simulink model "svpwm_2level_using_function"  (R2023a)
settings: Solver=VariableStepAuto  StartTime=0.0  StopTime=0.5  RelTol=1e-3
libraries: spsIGBTDiodeLib x6, spsVoltageMeasurementLib x5, spsSeriesRLCBranchLib x3, simulink x1, spsabctoAlphaBetaZeroLib x1, spsDCVoltageSourceLib x1, spsGroundLib x1, sps_lib x1
settings Model: Creator=yadur  LastModifiedBy=yadur

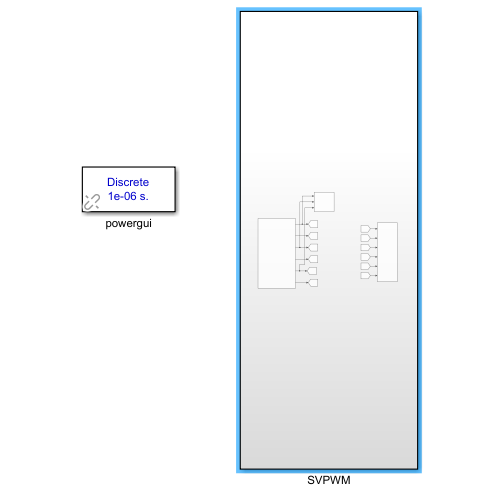
[thumbnail: Simulink's stored preview of the top-level diagram]
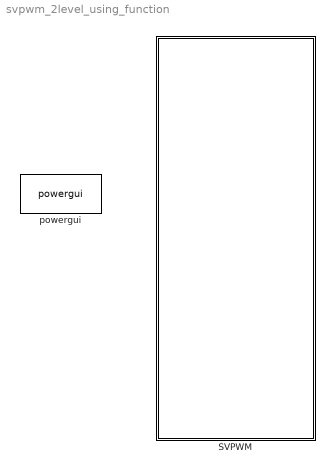
== system svpwm_2level_using_function ==
  SVPWM : Subsystem
  powergui : sps_lib/powergui  Priority=1  SimulationMode=Discrete  SampleTime=1e-6  frequency=60  Iterations=50  frequencyindice=0  Pbase=100e6  ErrMax=1e-4  UnitsV=kV  UnitsW=MW  buscounter=0  FunctionMessages=off  echomessages=off  EnableUseOfTLC=off  CurrentSourceSwitches=off  DisableSnubberDevices=off  DisableRonSwitches=off  DisableVfSwitches=off  DisplayEquations=off  AutomaticDiscreteSolvers=off  SolverType=Tustin/Backward Euler (TBE)  Interpol=off  ExternalGateDelay=off  methode=off  Ts=100  x0status=blocks  SPID=on  SwTol=0  HookPort=off  NonlinearTolerance=1e-4  nMaxIteration=100  ContinueOnMaxIteration=off  RestoreLinks=warning  ResistiveCurrentMeasurement=off  Frange=[0:2:500]  Ylog=off  Xlog=on  ShowGrid=off  save=off  variable=ZData  structure=0  ZoomFFT=off  StartTime=0.0  cycles=1  DisplayStyle=1  fundamental=60  FreqAxis=off  MaxFrequency=1000  frequencyindicesteady=1  RmsSteady=1  display=off

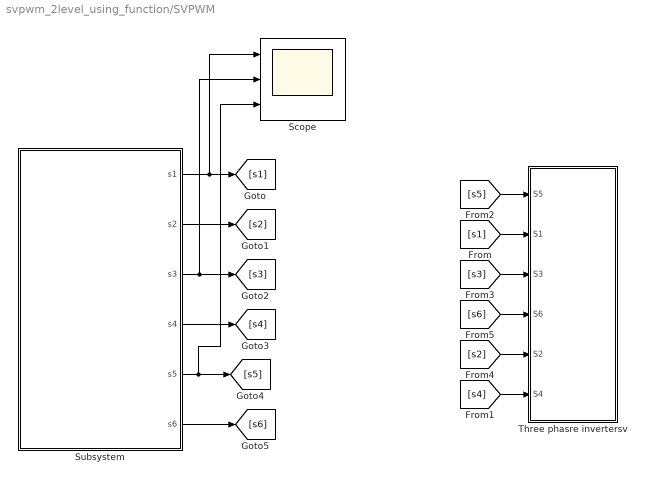
== system svpwm_2level_using_function/SVPWM ==
  Scope : Scope  NumInputPorts=3
  Subsystem : Subsystem
  Three phasre invertersv : Subsystem
  wires:
  [s1] -> Three phasre invertersv/2(S1)
  [s5] -> Three phasre invertersv/1(S5)
  [s3] -> Three phasre invertersv/3(S3)
  [s2] -> Three phasre invertersv/5(S2)
  Subsystem/6(s6) -> [s6]
  [s4] -> Three phasre invertersv/6(S4)
  Subsystem/5(s5) -> Scope/3, [s5]
  [s6] -> Three phasre invertersv/4(S6)
  Subsystem/1(s1) -> Scope/1, [s1]
  Subsystem/2(s2) -> [s2]
  Subsystem/4(s4) -> [s4]
  Subsystem/3(s3) -> Scope/2, [s3]

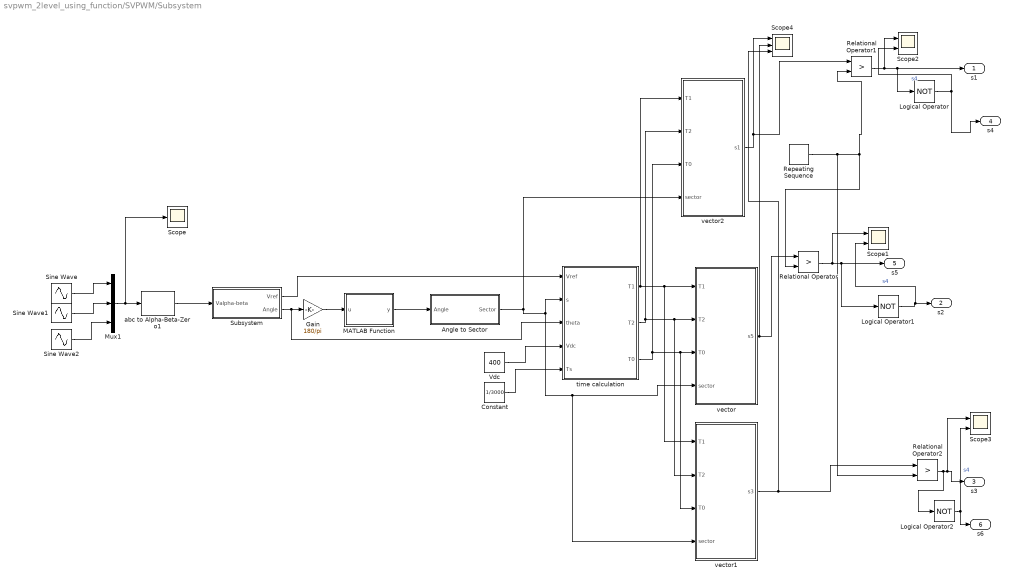
== system svpwm_2level_using_function/SVPWM/Subsystem ==
  Angle to Sector : Subsystem
  Constant : Constant  Value=1/3000
  Gain : Gain  Gain=180/pi
  Logical Operator : Logic  Operator=NOT  AllPortsSameDT=off  OutDataTypeStr=boolean
  Logical Operator1 : Logic  Operator=NOT  AllPortsSameDT=off  OutDataTypeStr=boolean
  Logical Operator2 : Logic  Operator=NOT  AllPortsSameDT=off  OutDataTypeStr=boolean
  MATLAB Function : MATLAB Function  TreatAsAtomicUnit=on
  Mux1 : Mux  Inputs=3
  Relational Operator : RelationalOperator  Operator=>  OutDataTypeStr=boolean  RndMeth=Simplest  InputSameDT=off
  Relational Operator1 : RelationalOperator  Operator=>  OutDataTypeStr=boolean  RndMeth=Simplest  InputSameDT=off
  Relational Operator2 : RelationalOperator  Operator=>  OutDataTypeStr=boolean  RndMeth=Simplest  InputSameDT=off
  Repeating Sequence : simulink/Sources/Repeating Sequence  rep_seq_t="[0  1]*[1/3000]"  rep_seq_y=[0 0.0025]
  Scope : Scope
  Scope1 : Scope  NumInputPorts=2
  Scope2 : Scope  NumInputPorts=2
  Scope3 : Scope  NumInputPorts=2
  Scope4 : Scope  NumInputPorts=3
  Sine Wave : Sin  Amplitude=230  Frequency=2*pi*50  SampleTime=0
  Sine Wave1 : Sin  Amplitude=230  Frequency=2*pi*50  Phase=2*pi/3  SampleTime=0
  Sine Wave2 : Sin  Amplitude=230  Frequency=2*pi*50  Phase=4*pi/3  SampleTime=0
  Subsystem : Subsystem
  Vdc : Constant  Value=400
  abc to Alpha-Beta-Zero1 : spsabctoAlphaBetaZeroLib/abc to Alpha-Beta-Zero
  time calculation : MATLAB Function  TreatAsAtomicUnit=on
  vector : MATLAB Function  TreatAsAtomicUnit=on
  vector1 : MATLAB Function  TreatAsAtomicUnit=on
  vector2 : MATLAB Function  TreatAsAtomicUnit=on
  s1 : Outport
  s2 : Outport  Port=2
  s3 : Outport  Port=3
  s4 : Outport  Port=4
  s5 : Outport  Port=5
  s6 : Outport  Port=6
  wires:
  Angle to Sector/1(Sector) -> vector1/4(sector), vector/4(sector), time calculation/2(s), vector2/4(sector)
  Sine Wave1/1 -> Mux1/2
  abc to Alpha-Beta-Zero1/1 -> Subsystem/1(Valpha-beta)
  Mux1/1 -> Scope/1, abc to Alpha-Beta-Zero1/1
  Vdc/1 -> time calculation/4(Vdc)
  Sine Wave/1 -> Mux1/1
  time calculation/3(T0) -> vector2/3(T0), vector1/3(T0), vector/3(T0)
  time calculation/1(T1) -> vector2/1(T1), vector1/1(T1), vector/1(T1)
  time calculation/2(T2) -> vector1/2(T2), vector/2(T2), vector2/2(T2)
  Logical Operator/1 -> s4/1, Scope2/2  "s4"
  Sine Wave2/1 -> Mux1/3
  vector/1(s5) -> Scope4/2, Relational Operator/1
  Relational Operator/1 -> Scope1/1, Logical Operator1/1, s5/1
  Relational Operator1/1 -> Scope2/1, Logical Operator/1, s1/1
  vector2/1(s1) -> Scope4/1, Relational Operator1/1
  Repeating Sequence/1 -> Relational Operator2/2, Relational Operator1/2, Relational Operator/2
  Relational Operator2/1 -> Logical Operator2/1, Scope3/1, s3/1
  vector1/1(s3) -> Scope4/3, Relational Operator2/1
  Logical Operator1/1 -> Scope1/2, s2/1  "s4"
  Logical Operator2/1 -> s6/1, Scope3/2  "s4"
  Constant/1 -> time calculation/5(Ts)
  Subsystem/1(Vref) -> time calculation/1(Vref)
  Subsystem/2(Angle) -> time calculation/3(theta), Gain/1
  Gain/1 -> MATLAB Function/1(u)
  MATLAB Function/1(y) -> Angle to Sector/1(Angle)

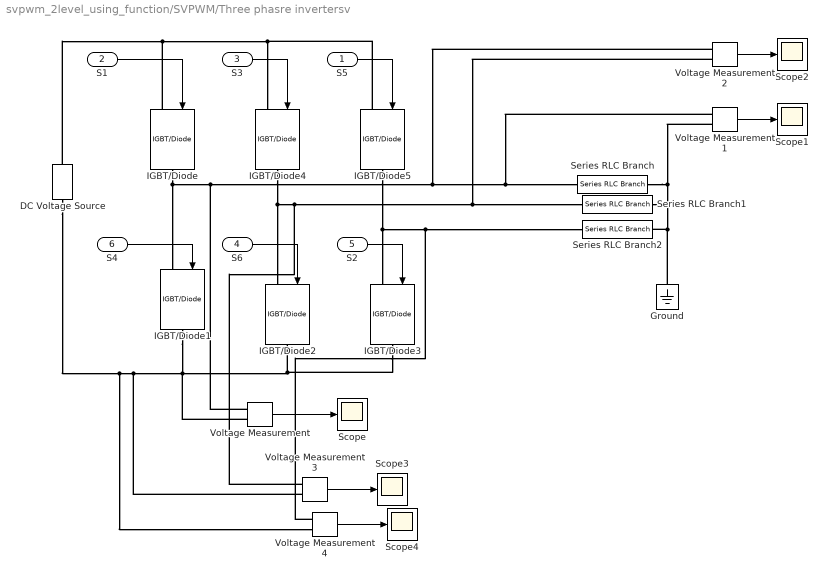
== system svpwm_2level_using_function/SVPWM/Three phasre invertersv ==
  S5 : Inport
  S1 : Inport  Port=2
  S3 : Inport  Port=3
  S6 : Inport  Port=4
  S2 : Inport  Port=5
  S4 : Inport  Port=6
  DC Voltage Source : spsDCVoltageSourceLib/DC Voltage Source  Amplitude=400  Measurements=None
  Ground : spsGroundLib/Ground  LConnTagsString=a
  IGBT/Diode{,1..5} (6 alike) : spsIGBTDiodeLib/IGBT//Diode  Ron=1e-3  Rs=1e5  Cs=inf  Measurements=off
  Scope{,1..4} (5 alike) : Scope
  Series RLC Branch : spsSeriesRLCBranchLib/Series RLC Branch  LConnTagsString=__new0  RConnTagsString=__new0  BranchType=R  Resistance=1  Inductance=1e-3  SetiL0=off  InitialCurrent=0  Capacitance=1e-6  Setx0=off  InitialVoltage=0  Measurements=None
  Series RLC Branch1 : spsSeriesRLCBranchLib/Series RLC Branch  LConnTagsString=__new0  RConnTagsString=__new0  BranchType=R  Resistance=1  Inductance=1e-3  SetiL0=off  InitialCurrent=0  Capacitance=1e-6  Setx0=off  InitialVoltage=0  Measurements=None
  Series RLC Branch2 : spsSeriesRLCBranchLib/Series RLC Branch  LConnTagsString=__new0  RConnTagsString=__new0  BranchType=R  Resistance=1  Inductance=1e-3  SetiL0=off  InitialCurrent=0  Capacitance=1e-6  Setx0=off  InitialVoltage=0  Measurements=None
  Voltage Measurement{,1..4} (5 alike) : spsVoltageMeasurementLib/Voltage Measurement  PhasorSimulation=off  OutputType=Complex  PSBequivalent=0
  wires:
  Voltage Measurement1/1 -> Scope1/1
  Voltage Measurement/1 -> Scope/1
  Voltage Measurement2/1 -> Scope2/1
  S3/1 -> IGBT/Diode4/1
  S5/1 -> IGBT/Diode5/1
  S2/1 -> IGBT/Diode3/1
  S4/1 -> IGBT/Diode1/1
  S6/1 -> IGBT/Diode2/1
  S1/1 -> IGBT/Diode/1
  Voltage Measurement3/1 -> Scope3/1
  Voltage Measurement4/1 -> Scope4/1
  connections:
  IGBT/Diode3/RConn1 -- IGBT/Diode2/RConn1 -- Voltage Measurement3/LConn2 -- Voltage Measurement4/LConn2 -- DC Voltage Source/LConn1 -- Voltage Measurement/LConn2 -- IGBT/Diode1/RConn1
  IGBT/Diode5/RConn1 -- IGBT/Diode3/LConn1 -- Voltage Measurement4/LConn1 -- Series RLC Branch2/LConn1
  IGBT/Diode5/LConn1 -- DC Voltage Source/RConn1 -- IGBT/Diode/LConn1 -- IGBT/Diode4/LConn1
  IGBT/Diode4/RConn1 -- IGBT/Diode2/LConn1 -- Voltage Measurement3/LConn1 -- Voltage Measurement2/LConn2 -- Series RLC Branch1/LConn1
  IGBT/Diode/RConn1 -- Voltage Measurement/LConn1 -- Voltage Measurement2/LConn1 -- Voltage Measurement1/LConn1 -- Series RLC Branch/LConn1 -- IGBT/Diode1/LConn1
  Series RLC Branch/RConn1 -- Ground/LConn1 -- Series RLC Branch2/RConn1 -- Series RLC Branch1/RConn1 -- Voltage Measurement1/LConn2

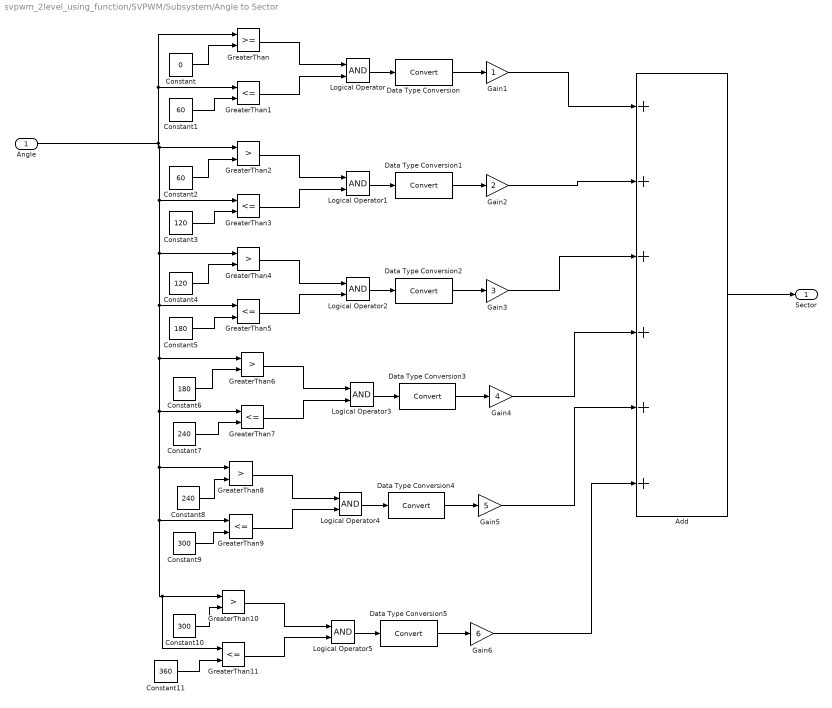
== system svpwm_2level_using_function/SVPWM/Subsystem/Angle to Sector ==
  Angle : Inport
  Add : Sum  Inputs=++++++
  Constant : Constant  Value=0
  Constant1 : Constant  Value=60
  Constant10 : Constant  Value=300
  Constant11 : Constant  Value=360
  Constant2 : Constant  Value=60
  Constant3 : Constant  Value=120
  Constant4 : Constant  Value=120
  Constant5 : Constant  Value=180
  Constant6 : Constant  Value=180
  Constant7 : Constant  Value=240
  Constant8 : Constant  Value=240
  Constant9 : Constant  Value=300
  Data Type Conversion{,1..5} (6 alike) : DataTypeConversion  SaturateOnIntegerOverflow=off  RndMeth=Floor
  Gain1 : Gain
  Gain2 : Gain  Gain=2
  Gain3 : Gain  Gain=3
  Gain4 : Gain  Gain=4
  Gain5 : Gain  Gain=5
  Gain6 : Gain  Gain=6
  GreaterThan : RelationalOperator  OutDataTypeStr=boolean  RndMeth=Simplest  InputSameDT=off
  GreaterThan{1,3,5,7,9,11} (6 alike) : RelationalOperator  Operator=<=  OutDataTypeStr=boolean  RndMeth=Simplest  InputSameDT=off
  GreaterThan{2,4,6,8,10} (5 alike) : RelationalOperator  Operator=>  OutDataTypeStr=boolean  RndMeth=Simplest  InputSameDT=off
  Logical Operator{,1..5} (6 alike) : Logic  AllPortsSameDT=off  OutDataTypeStr=boolean
  Sector : Outport
  wires:
  Constant/1 -> GreaterThan/2
  Constant1/1 -> GreaterThan1/2
  GreaterThan/1 -> Logical Operator/1
  GreaterThan1/1 -> Logical Operator/2
  Logical Operator/1 -> Data Type Conversion/1
  Data Type Conversion/1 -> Gain1/1
  GreaterThan2/1 -> Logical Operator1/1
  Data Type Conversion1/1 -> Gain2/1
  Constant3/1 -> GreaterThan3/2
  Constant2/1 -> GreaterThan2/2
  GreaterThan3/1 -> Logical Operator1/2
  Logical Operator1/1 -> Data Type Conversion1/1
  GreaterThan4/1 -> Logical Operator2/1
  Data Type Conversion2/1 -> Gain3/1
  Constant5/1 -> GreaterThan5/2
  Constant4/1 -> GreaterThan4/2
  GreaterThan5/1 -> Logical Operator2/2
  Logical Operator2/1 -> Data Type Conversion2/1
  GreaterThan6/1 -> Logical Operator3/1
  Data Type Conversion3/1 -> Gain4/1
  Constant7/1 -> GreaterThan7/2
  Constant6/1 -> GreaterThan6/2
  GreaterThan7/1 -> Logical Operator3/2
  Logical Operator3/1 -> Data Type Conversion3/1
  GreaterThan8/1 -> Logical Operator4/1
  Data Type Conversion4/1 -> Gain5/1
  Constant9/1 -> GreaterThan9/2
  Constant8/1 -> GreaterThan8/2
  GreaterThan9/1 -> Logical Operator4/2
  Logical Operator4/1 -> Data Type Conversion4/1
  GreaterThan10/1 -> Logical Operator5/1
  Data Type Conversion5/1 -> Gain6/1
  Constant11/1 -> GreaterThan11/2
  Constant10/1 -> GreaterThan10/2
  GreaterThan11/1 -> Logical Operator5/2
  Logical Operator5/1 -> Data Type Conversion5/1
  Angle/1 -> GreaterThan11/1, GreaterThan10/1, GreaterThan9/1, GreaterThan8/1, GreaterThan7/1, GreaterThan6/1, GreaterThan5/1, GreaterThan4/1, GreaterThan3/1, GreaterThan2/1, GreaterThan1/1, GreaterThan/1
  Gain1/1 -> Add/1
  Gain2/1 -> Add/2
  Gain3/1 -> Add/3
  Gain4/1 -> Add/4
  Gain5/1 -> Add/5
  Gain6/1 -> Add/6
  Add/1 -> Sector/1

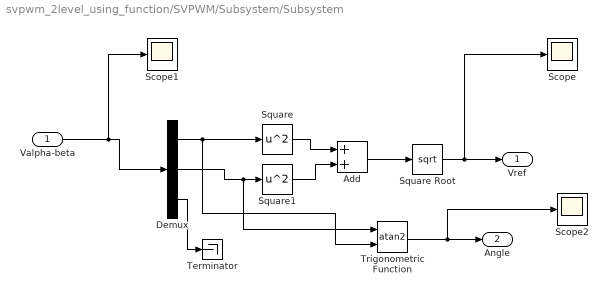
== system svpwm_2level_using_function/SVPWM/Subsystem/Subsystem ==
  Valpha-beta : Inport
  Add : Sum
  Demux : Demux  Outputs=3
  Scope : Scope
  Scope1 : Scope
  Scope2 : Scope
  Square : Math  Operator=square
  Square Root : Sqrt
  Square1 : Math  Operator=square
  Terminator : Terminator
  Trigonometric Function : Trigonometry  Operator=atan2
  Vref : Outport
  Angle : Outport  Port=2
  wires:
  Valpha-beta/1 -> Scope1/1, Demux/1
  Demux/3 -> Terminator/1
  Demux/1 -> Trigonometric Function/2, Square/1
  Demux/2 -> Trigonometric Function/1, Square1/1
  Square/1 -> Add/1
  Square1/1 -> Add/2
  Add/1 -> Square Root/1
  Square Root/1 -> Scope/1, Vref/1
  Trigonometric Function/1 -> Scope2/1, Angle/1

== matlab function svpwm_2level_using_function/SVPWM/Subsystem/vector1 ==
  data: T1 input; T2 input; T0 input; sector input; s3 output
function s3  = fcn(T1,T2,T0,sector)

s3=0;

if(sector==4 || sector==5)
s3=T1+T2+T0/2 ;   
    
elseif(sector==6)


     s3=T1+T0/2 ;
     

elseif(sector==1 || sector==2)

s3=T0/2  ;

  


elseif(sector==3)

 s3=T2+T0/2  ;                    

              

 
end

== matlab function svpwm_2level_using_function/SVPWM/Subsystem/vector2 ==
  data: T1 input; T2 input; T0 input; sector input; s1 output
function s1  = fcn(T1,T2,T0,sector)
 s1=0 ;

if(sector==1 || sector==6)
s1=T1+T2+T0/2 ;
    
elseif(sector==2)
 s1=T1+T0/2 ;
     

elseif(sector==3 ||sector==4)

s1=T0/2  ;
elseif(sector==5)
s1=T2+T0/2  ;                    


        
end

== matlab function svpwm_2level_using_function/SVPWM/Subsystem/MATLAB Function ==
  data: u input; y output
function y = fcn(u)

angle=u(1);

if(angle > 0)
    y=angle;
else 
    y=angle + 360;

end
end

== matlab function svpwm_2level_using_function/SVPWM/Subsystem/time calculation ==
  data: Vref input; T1 output; s input; theta input; Vdc input; T2 output; T0 output; Ts input
function [T1,T2,T0] = fcn(Vref,s,theta,Vdc,Ts)

ma=sqrt(3)*Ts*Vref/Vdc ;
T1=ma*sin(s*pi/3 - theta);
T2=ma*sin(-(s-1)*pi/3 + theta);
T0=Ts-T1-T2;
end

== matlab function svpwm_2level_using_function/SVPWM/Subsystem/vector ==
  data: T1 input; T2 input; T0 input; sector input; s5 output
function s5  = fcn(T1,T2,T0,sector)

s5=0 ;


if(sector==2 || sector==3)
s5=T1+T2+T0/2 ;


              


    
    
elseif(sector==4)


     s5=T1+T0/2 ;
     

elseif(sector==5 || sector==6)

s5=T0/2  ;

  


elseif(sector==1)

 s5=T2+T0/2  ;                    

              

 
end
